simulink model "untitled"  (R2021a)
settings: Solver=VariableStepAuto  StartTime=0.0  StopTime=10.0  RelTol=1e-3
settings Model: Creator=Jakob Gammelgaard  LastModifiedBy=Jakob Gammelgaard

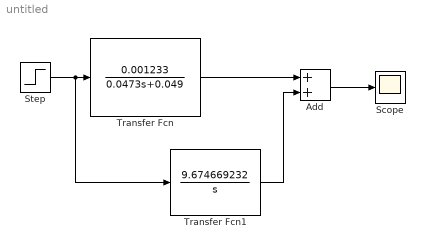
== system untitled ==
  Add : Sum
  Scope : Scope
  Step : Step  SampleTime=0
  Transfer Fcn : TransferFcn  Numerator=[0.001233]  Denominator=[0.0473 0.049]
  Transfer Fcn1 : TransferFcn  Numerator=[9.674669232]  Denominator=[1 0]
  wires:
  Transfer Fcn/1 -> Add/1
  Transfer Fcn1/1 -> Add/2
  Step/1 -> Transfer Fcn1/1, Transfer Fcn/1
  Add/1 -> Scope/1
